simulink model "AntiWindupSim"  (R2020b)
settings: Solver=ode45  StartTime=0.0  StopTime=9  RelTol=1e-3
values from neighbouring files (symbols this model uses):
  BEMFCompGain = N*Ke/Kdrv    [AntiWindup_Feed_FWD.m]
  frictionCompGain = Req / (Kdrv*Kt*N)    [AntiWindup_Feed_FWD.m]
  inertiaCompGain = N*Req*Jeq_est/(Kdrv*Kt)    [AntiWindup_Feed_FWD.m]
  Kw = 1/Tw    [AntiWindup_Feed_FWD.m]
  tausf = tausf_est    [FromEstimationToSet.m]
undefined symbols (not defined in the file or in its folder): Beq_est, deg2pulse, Kd, Kdrv, Ke, Keq, Ki, Kmot, Kp, Kt, N, pulse2deg, rad2rpm, rpm2degs, tausf_est, Tdrv, Teq, Tl, Tmot, Tsample, vcc, vdd, vm, vp
libraries: simulink x2
settings Model: Creator=Utente  LastModifiedBy=Utente
settings SolverCC: ZeroCrossAlgorithm=Adaptive
settings DebuggingCC: IgnoredZcDiagnostic=none

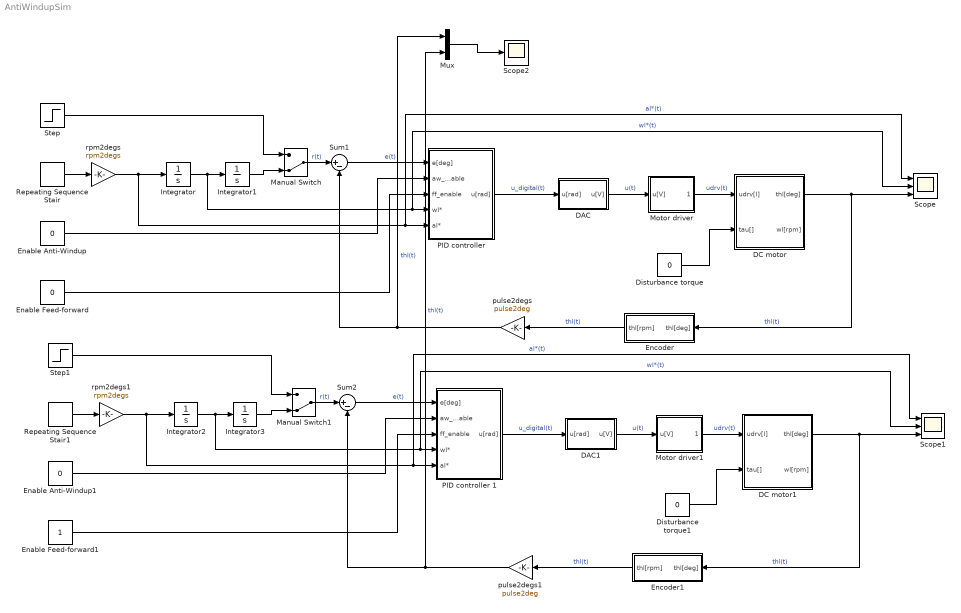
== system AntiWindupSim ==
  DAC : Subsystem
  DAC1 : Subsystem
  DC motor : Subsystem
  DC motor1 : Subsystem
  Disturbance torque : Constant  Value=0
  Disturbance torque1 : Constant  Value=0
  Enable Anti-Windup : Constant  Value=0
  Enable Anti-Windup1 : Constant  Value=0
  Enable Feed-forward : Constant  Value=0
  Enable Feed-forward1 : Constant
  Encoder : Subsystem
  Encoder1 : Subsystem
  Integrator{,1..3} (4 alike) : Integrator
  Manual Switch : ManualSwitch  CurrentSetting=0
  Manual Switch1 : ManualSwitch  CurrentSetting=0
  Motor driver : Subsystem
  Motor driver1 : Subsystem
  Mux : Mux  Inputs=2
  "PID controller " : Subsystem
  PID controller 1 : Subsystem
  Repeating Sequence Stair : simulink/Sources/Repeating Sequence Stair  OutValues=[900 0 -900 -900 0 900].'  tsamp=0.5  OutMin=[]  OutMax=[]  OutDataTypeStr=double  OutputDataTypeScalingMode=double  OutDataType=fixdt(0,8)  ConRadixGroup=Best Precision: Vector-wise  OutScaling=2^-12
  Repeating Sequence Stair1 : simulink/Sources/Repeating Sequence Stair  OutValues=[900 0 -900 -900 0 900].'  tsamp=0.5  OutMin=[]  OutMax=[]  OutDataTypeStr=double  OutputDataTypeScalingMode=double  OutDataType=fixdt(0,8)  ConRadixGroup=Best Precision: Vector-wise  OutScaling=2^-12
  Scope : Scope  NumInputPorts=3
  Scope1 : Scope  NumInputPorts=3
  Scope2 : Scope
  Step : Step  Time=0  After=360  SampleTime=0
  Step1 : Step  Time=0  After=360  SampleTime=0
  Sum1 : Sum  Inputs=|+-
  Sum2 : Sum  Inputs=|+-
  pulse2degs : Gain  Gain=pulse2deg
  pulse2degs1 : Gain  Gain=pulse2deg
  rpm2degs : Gain  Gain=rpm2degs
  rpm2degs1 : Gain  Gain=rpm2degs
  wires:
  Motor driver/1(udrv[I]) -> DC motor/1(udrv[I])  "udrv(t)"
  DAC/1(u[V]) -> Motor driver/1(u[V])  "u(t)"
  Encoder/1(thl[rpm]) -> pulse2degs/1  "thl(t)"
  pulse2degs/1 -> Sum1/2, Mux/1  "thl(t)"
  Sum1/1 -> "PID controller "/1(e[deg])  "e(t)"
  "PID controller "/1(u[rad]) -> DAC/1(u[rad])  "u_digital(t)"
  DC motor/1(thl[deg]) -> Scope/3, Encoder/1(thl[deg])  "thl(t)"
  Step/1 -> Manual Switch/1
  Disturbance torque/1 -> DC motor/2(tau[])
  Enable Anti-Windup/1 -> "PID controller "/2(aw_enable)
  Manual Switch/1 -> Sum1/1  "r(t)"
  Enable Feed-forward/1 -> "PID controller "/3(ff_enable)
  Repeating Sequence Stair/1 -> rpm2degs/1
  rpm2degs/1 -> Scope/1, "PID controller "/5(al*), Integrator/1  "al*(t)"
  Integrator1/1 -> Manual Switch/2
  Integrator/1 -> Scope/2, "PID controller "/4(wl*), Integrator1/1  "wl*(t)"
  Encoder1/1(thl[rpm]) -> pulse2degs1/1  "thl(t)"
  Repeating Sequence Stair1/1 -> rpm2degs1/1
  Enable Anti-Windup1/1 -> PID controller 1/2(aw_enable)
  Integrator3/1 -> Manual Switch1/2
  Enable Feed-forward1/1 -> PID controller 1/3(ff_enable)
  Disturbance torque1/1 -> DC motor1/2(tau[])
  Manual Switch1/1 -> Sum2/1  "r(t)"
  Step1/1 -> Manual Switch1/1
  DC motor1/1(thl[deg]) -> Scope1/3, Encoder1/1(thl[deg])  "thl(t)"
  Sum2/1 -> PID controller 1/1(e[deg])  "e(t)"
  Integrator2/1 -> Scope1/2, PID controller 1/4(wl*), Integrator3/1  "wl*(t)"
  DAC1/1(u[V]) -> Motor driver1/1(u[V])  "u(t)"
  Motor driver1/1(udrv[I]) -> DC motor1/1(udrv[I])  "udrv(t)"
  rpm2degs1/1 -> Scope1/1, PID controller 1/5(al*), Integrator2/1  "al*(t)"
  pulse2degs1/1 -> Sum2/2, Mux/2  "thl(t)"
  PID controller 1/1(u[rad]) -> DAC1/1(u[rad])  "u_digital(t)"
  Mux/1 -> Scope2/1

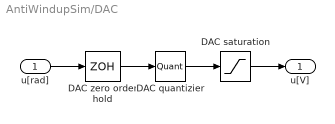
== system AntiWindupSim/DAC ==
  u[rad] : Inport
  DAC quantizier : Quantizer  QuantizationInterval=q_step
  DAC saturation : Saturate  UpperLimit=vdd  LowerLimit=vcc
  DAC zero order hold : ZeroOrderHold  SampleTime=Tsample
  u[V] : Outport
  wires:
  DAC quantizier/1 -> DAC saturation/1
  DAC zero order hold/1 -> DAC quantizier/1
  DAC saturation/1 -> u[V]/1
  u[rad]/1 -> DAC zero order hold/1

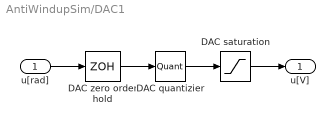
== system AntiWindupSim/DAC1 ==
  u[rad] : Inport
  DAC quantizier : Quantizer  QuantizationInterval=q_step
  DAC saturation : Saturate  UpperLimit=vdd  LowerLimit=vcc
  DAC zero order hold : ZeroOrderHold  SampleTime=Tsample
  u[V] : Outport
  wires:
  DAC quantizier/1 -> DAC saturation/1
  DAC zero order hold/1 -> DAC quantizier/1
  DAC saturation/1 -> u[V]/1
  u[rad]/1 -> DAC zero order hold/1

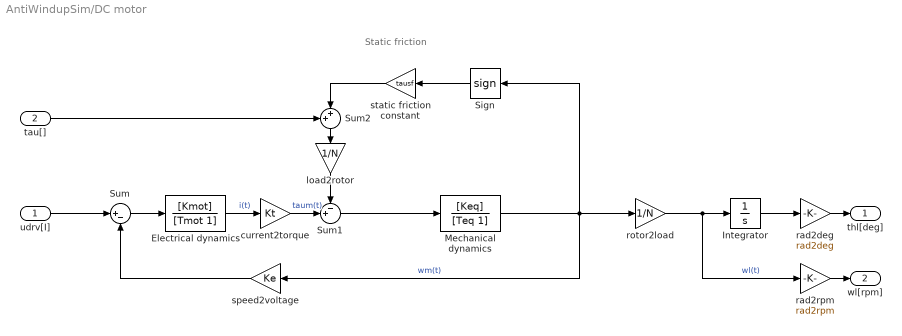
== system AntiWindupSim/DC motor ==
  note: Static friction
  udrv[I] : Inport  Unit=V
  tau[] : Inport  Port=2  Unit=V
  Electrical dynamics : TransferFcn  Numerator=[Kmot]  Denominator=[Tmot 1]
  Integrator : Integrator
  Mechanical dynamics : TransferFcn  Numerator=[Keq]  Denominator=[Teq 1]
  Sign : Signum  ZeroCross=off
  Sum : Sum  Inputs=|+-
  Sum1 : Sum  Inputs=-+|
  Sum2 : Sum  Inputs=++|
  current2torque : Gain  Gain=Kt
  load2rotor : Gain  Gain=1/N
  rad2deg : Gain  Gain=rad2deg
  rad2rpm : Gain  Gain=rad2rpm
  rotor2load : Gain  Gain=1/N
  speed2voltage : Gain  Gain=Ke
  static friction constant : Gain  Gain=tausf
  thl[deg] : Outport  Unit=deg
  wl[rpm] : Outport  Port=2  Unit=rpm
  wires:
  load2rotor/1 -> Sum1/1
  Mechanical dynamics/1 -> Sign/1, rotor2load/1, speed2voltage/1  "wm(t)"
  Sign/1 -> static friction constant/1
  current2torque/1 -> Sum1/2  "taum(t)"
  Sum1/1 -> Mechanical dynamics/1
  speed2voltage/1 -> Sum/2
  rotor2load/1 -> rad2rpm/1, Integrator/1  "wl(t)"
  Electrical dynamics/1 -> current2torque/1  "i(t)"
  Integrator/1 -> rad2deg/1
  Sum/1 -> Electrical dynamics/1
  rad2rpm/1 -> wl[rpm]/1
  rad2deg/1 -> thl[deg]/1
  udrv[I]/1 -> Sum/1
  static friction constant/1 -> Sum2/2
  Sum2/1 -> load2rotor/1
  tau[]/1 -> Sum2/1

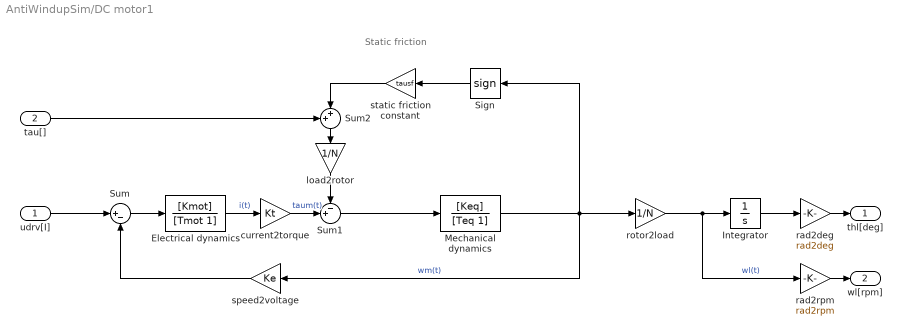
== system AntiWindupSim/DC motor1 ==
  note: Static friction
  udrv[I] : Inport  Unit=V
  tau[] : Inport  Port=2  Unit=V
  Electrical dynamics : TransferFcn  Numerator=[Kmot]  Denominator=[Tmot 1]
  Integrator : Integrator
  Mechanical dynamics : TransferFcn  Numerator=[Keq]  Denominator=[Teq 1]
  Sign : Signum  ZeroCross=off
  Sum : Sum  Inputs=|+-
  Sum1 : Sum  Inputs=-+|
  Sum2 : Sum  Inputs=++|
  current2torque : Gain  Gain=Kt
  load2rotor : Gain  Gain=1/N
  rad2deg : Gain  Gain=rad2deg
  rad2rpm : Gain  Gain=rad2rpm
  rotor2load : Gain  Gain=1/N
  speed2voltage : Gain  Gain=Ke
  static friction constant : Gain  Gain=tausf
  thl[deg] : Outport  Unit=deg
  wl[rpm] : Outport  Port=2  Unit=rpm
  wires:
  load2rotor/1 -> Sum1/1
  Mechanical dynamics/1 -> Sign/1, rotor2load/1, speed2voltage/1  "wm(t)"
  Sign/1 -> static friction constant/1
  current2torque/1 -> Sum1/2  "taum(t)"
  Sum1/1 -> Mechanical dynamics/1
  speed2voltage/1 -> Sum/2
  rotor2load/1 -> rad2rpm/1, Integrator/1  "wl(t)"
  Electrical dynamics/1 -> current2torque/1  "i(t)"
  Integrator/1 -> rad2deg/1
  Sum/1 -> Electrical dynamics/1
  rad2rpm/1 -> wl[rpm]/1
  rad2deg/1 -> thl[deg]/1
  udrv[I]/1 -> Sum/1
  static friction constant/1 -> Sum2/2
  Sum2/1 -> load2rotor/1
  tau[]/1 -> Sum2/1

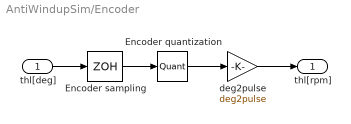
== system AntiWindupSim/Encoder ==
  thl[deg] : Inport
  Encoder quantization : Quantizer  QuantizationInterval=enc_step
  Encoder sampling : ZeroOrderHold  SampleTime=Tsample
  deg2pulse : Gain  Gain=deg2pulse
  thl[rpm] : Outport
  wires:
  Encoder quantization/1 -> deg2pulse/1
  deg2pulse/1 -> thl[rpm]/1
  Encoder sampling/1 -> Encoder quantization/1
  thl[deg]/1 -> Encoder sampling/1

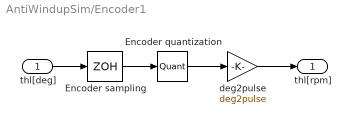
== system AntiWindupSim/Encoder1 ==
  thl[deg] : Inport
  Encoder quantization : Quantizer  QuantizationInterval=enc_step
  Encoder sampling : ZeroOrderHold  SampleTime=Tsample
  deg2pulse : Gain  Gain=deg2pulse
  thl[rpm] : Outport
  wires:
  Encoder quantization/1 -> deg2pulse/1
  deg2pulse/1 -> thl[rpm]/1
  Encoder sampling/1 -> Encoder quantization/1
  thl[deg]/1 -> Encoder sampling/1

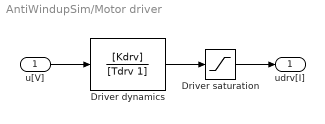
== system AntiWindupSim/Motor driver ==
  u[V] : Inport
  Driver dynamics : TransferFcn  Numerator=[Kdrv]  Denominator=[Tdrv 1]
  Driver saturation : Saturate  UpperLimit=vp  LowerLimit=vm
  udrv[I] : Outport
  wires:
  Driver saturation/1 -> udrv[I]/1
  Driver dynamics/1 -> Driver saturation/1
  u[V]/1 -> Driver dynamics/1

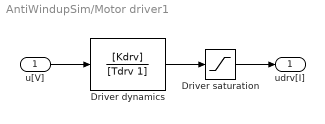
== system AntiWindupSim/Motor driver1 ==
  u[V] : Inport
  Driver dynamics : TransferFcn  Numerator=[Kdrv]  Denominator=[Tdrv 1]
  Driver saturation : Saturate  UpperLimit=vp  LowerLimit=vm
  udrv[I] : Outport
  wires:
  Driver saturation/1 -> udrv[I]/1
  Driver dynamics/1 -> Driver saturation/1
  u[V]/1 -> Driver dynamics/1

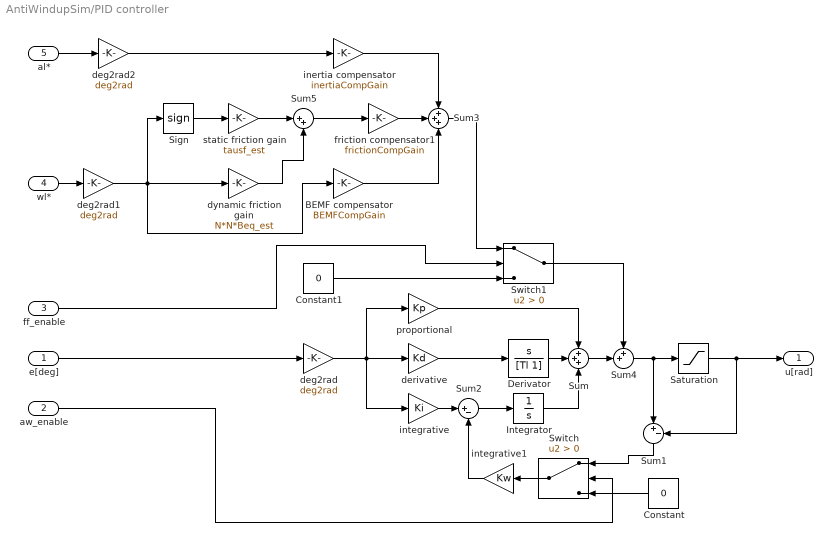
== system AntiWindupSim/PID controller  ==
  e[deg] : Inport  Unit=deg
  aw_enable : Inport  Port=2  Unit=deg
  ff_enable : Inport  Port=3  Unit=deg
  wl* : Inport  Port=4  Unit=deg
  al* : Inport  Port=5  Unit=deg
  BEMF compensator : Gain  Gain=BEMFCompGain
  Constant : Constant  Value=0
  Constant1 : Constant  Value=0
  Derivator : TransferFcn  Numerator=[1 0]  Denominator=[Tl 1]
  Integrator : Integrator
  Saturation : Saturate  UpperLimit=vdd  LowerLimit=vcc
  Sign : Signum
  Sum : Sum  Inputs=+++
  Sum1 : Sum  Inputs=|+-
  Sum2 : Sum  Inputs=|+-
  Sum3 : Sum  Inputs=+++
  Sum4 : Sum  Inputs=++|
  Sum5 : Sum  Inputs=|++
  Switch : Switch  Criteria=u2 > Threshold
  Switch1 : Switch  Criteria=u2 > Threshold
  deg2rad : Gain  Gain=deg2rad
  deg2rad1 : Gain  Gain=deg2rad
  deg2rad2 : Gain  Gain=deg2rad
  derivative : Gain  Gain=Kd
  dynamic friction gain : Gain  Gain=N*N*Beq_est
  friction compensator1 : Gain  Gain=frictionCompGain
  inertia compensator : Gain  Gain=inertiaCompGain
  integrative : Gain  Gain=Ki
  integrative1 : Gain  Gain=Kw
  proportional : Gain  Gain=Kp
  static friction gain : Gain  Gain=tausf_est
  u[rad] : Outport
  wires:
  e[deg]/1 -> deg2rad/1
  deg2rad/1 -> integrative/1, derivative/1, proportional/1
  proportional/1 -> Sum/1
  Saturation/1 -> Sum1/2, u[rad]/1
  integrative/1 -> Sum2/1
  Sum2/1 -> Integrator/1
  integrative1/1 -> Sum2/2
  Integrator/1 -> Sum/3
  Derivator/1 -> Sum/2
  derivative/1 -> Derivator/1
  aw_enable/1 -> Switch/2
  Constant/1 -> Switch/3
  Switch/1 -> integrative1/1
  Sum1/1 -> Switch/1
  ff_enable/1 -> Switch1/2
  Constant1/1 -> Switch1/3
  friction compensator1/1 -> Sum3/2
  inertia compensator/1 -> Sum3/1
  BEMF compensator/1 -> Sum3/3
  Sum4/1 -> Sum1/1, Saturation/1
  Sign/1 -> static friction gain/1
  static friction gain/1 -> Sum5/1
  dynamic friction gain/1 -> Sum5/2
  Sum5/1 -> friction compensator1/1
  al*/1 -> deg2rad2/1
  wl*/1 -> deg2rad1/1
  Sum3/1 -> Switch1/1
  Sum/1 -> Sum4/2
  Switch1/1 -> Sum4/1
  deg2rad1/1 -> BEMF compensator/1, Sign/1, dynamic friction gain/1
  deg2rad2/1 -> inertia compensator/1

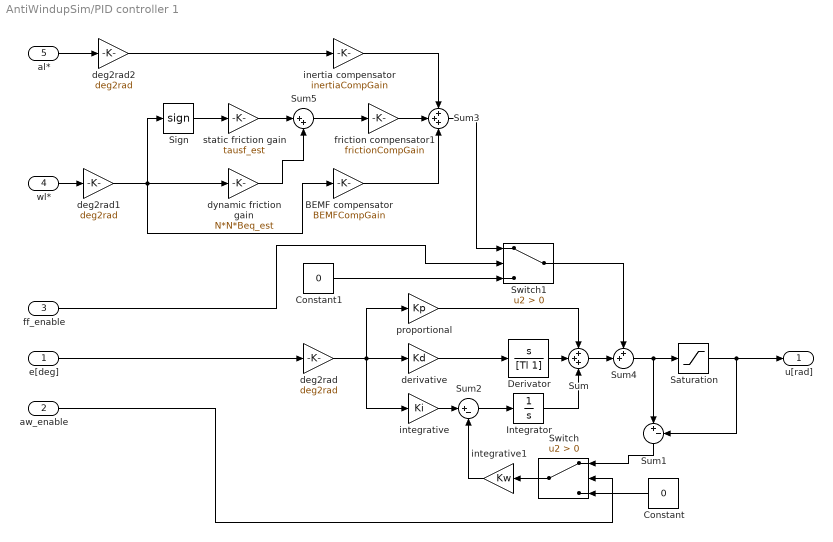
== system AntiWindupSim/PID controller 1 ==
  e[deg] : Inport  Unit=deg
  aw_enable : Inport  Port=2  Unit=deg
  ff_enable : Inport  Port=3  Unit=deg
  wl* : Inport  Port=4  Unit=deg
  al* : Inport  Port=5  Unit=deg
  BEMF compensator : Gain  Gain=BEMFCompGain
  Constant : Constant  Value=0
  Constant1 : Constant  Value=0
  Derivator : TransferFcn  Numerator=[1 0]  Denominator=[Tl 1]
  Integrator : Integrator
  Saturation : Saturate  UpperLimit=vdd  LowerLimit=vcc
  Sign : Signum
  Sum : Sum  Inputs=+++
  Sum1 : Sum  Inputs=|+-
  Sum2 : Sum  Inputs=|+-
  Sum3 : Sum  Inputs=+++
  Sum4 : Sum  Inputs=++|
  Sum5 : Sum  Inputs=|++
  Switch : Switch  Criteria=u2 > Threshold
  Switch1 : Switch  Criteria=u2 > Threshold
  deg2rad : Gain  Gain=deg2rad
  deg2rad1 : Gain  Gain=deg2rad
  deg2rad2 : Gain  Gain=deg2rad
  derivative : Gain  Gain=Kd
  dynamic friction gain : Gain  Gain=N*N*Beq_est
  friction compensator1 : Gain  Gain=frictionCompGain
  inertia compensator : Gain  Gain=inertiaCompGain
  integrative : Gain  Gain=Ki
  integrative1 : Gain  Gain=Kw
  proportional : Gain  Gain=Kp
  static friction gain : Gain  Gain=tausf_est
  u[rad] : Outport
  wires:
  e[deg]/1 -> deg2rad/1
  deg2rad/1 -> integrative/1, derivative/1, proportional/1
  proportional/1 -> Sum/1
  Saturation/1 -> Sum1/2, u[rad]/1
  integrative/1 -> Sum2/1
  Sum2/1 -> Integrator/1
  integrative1/1 -> Sum2/2
  Integrator/1 -> Sum/3
  Derivator/1 -> Sum/2
  derivative/1 -> Derivator/1
  aw_enable/1 -> Switch/2
  Constant/1 -> Switch/3
  Switch/1 -> integrative1/1
  Sum1/1 -> Switch/1
  ff_enable/1 -> Switch1/2
  Constant1/1 -> Switch1/3
  friction compensator1/1 -> Sum3/2
  inertia compensator/1 -> Sum3/1
  BEMF compensator/1 -> Sum3/3
  Sum4/1 -> Sum1/1, Saturation/1
  Sign/1 -> static friction gain/1
  static friction gain/1 -> Sum5/1
  dynamic friction gain/1 -> Sum5/2
  Sum5/1 -> friction compensator1/1
  al*/1 -> deg2rad2/1
  wl*/1 -> deg2rad1/1
  Sum3/1 -> Switch1/1
  Sum/1 -> Sum4/2
  Switch1/1 -> Sum4/1
  deg2rad1/1 -> BEMF compensator/1, Sign/1, dynamic friction gain/1
  deg2rad2/1 -> inertia compensator/1
